simulink model "PID_controller"  (R2021a)
settings: Solver=VariableStepAuto  StartTime=0.0  StopTime=100  RelTol=1e-3
model workspace (MAT data in the model file):
  Kd = 230
  Ki = 120
  Kp = 1250
  N = 100000
settings Model: DataDictionary=data.sldd  Creator=znome  LastModifiedBy=AVM
settings SolverCC: AlgebraicLoopSolver=TrustRegion
settings DataIOCC: SaveOutput=off  SaveTime=off
settings DebuggingCC: SFMachineParentedDataDiag=warning
settings SimscapeCC: SimscapeNormalizeSystem=off

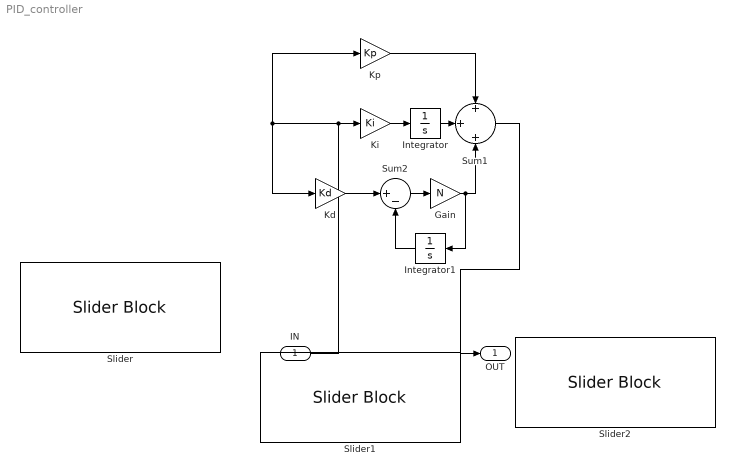
== system PID_controller ==
  IN : Inport  OutDataTypeStr=double  PortDimensions=1  SampleTime=0
  Gain : Gain  Gain=N
  Integrator : Integrator
  Integrator1 : Integrator
  Kd : Gain  Gain=Kd
  Ki : Gain  Gain=Ki
  Kp : Gain  Gain=Kp
  Slider : SliderBlock
  Slider1 : SliderBlock
  Slider2 : SliderBlock
  Sum1 : Sum  Inputs=+|+|+
  Sum2 : Sum  Inputs=|+-
  OUT : Outport  OutDataTypeStr=double  PortDimensions=1  SampleTime=0
  wires:
  IN/1 -> Ki/1, Kd/1, Kp/1
  Ki/1 -> Integrator/1
  Kd/1 -> Sum2/1
  Integrator/1 -> Sum1/2
  Kp/1 -> Sum1/1
  Sum2/1 -> Gain/1
  Sum1/1 -> OUT/1
  Gain/1 -> Integrator1/1, Sum1/3
  Integrator1/1 -> Sum2/2
